simulink model "Model_PID_pitch2010a"  (Simulink 8.9)
settings: Solver=ode45  StartTime=0.0  StopTime=100  RelTol=1e-3  EnableMultiTasking=on
libraries: fuzblock x1
settings Model: Creator=Eng mohammad dradkah  LastModifiedBy=Andres
settings OptimizationCC: ExpressionDepthLimit=2147483647  InitFltsAndDblsToZero=on
settings DebuggingCC: SaveWithParameterizedLinksMsg=none  SignalResolutionControl=TryResolveAllWithWarning  MultiTaskDSMMsg=warning  MultiTaskCondExecSysMsg=none
settings GRTTargetCC: TargetFcnLib=ansi_tfl_tmw.mat  GeneratePreprocessorConditionals=Use local settings

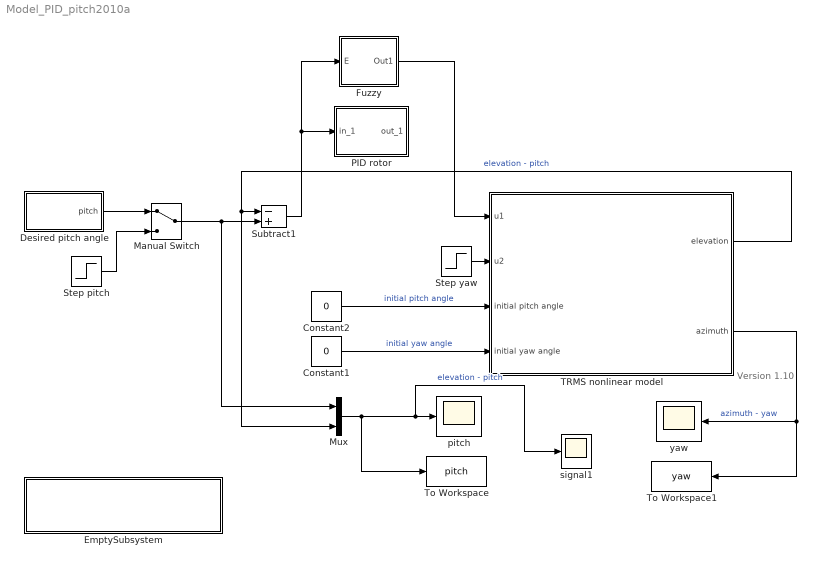
== system Model_PID_pitch2010a ==
  note: Version 1.10
  Constant1 : Constant  Value=0
  Constant2 : Constant  Value=0
  Desired pitch angle : Subsystem
  EmptySubsystem : Subsystem
      mask Display:
      | image(imread('FB-inst-blue2.jpg'))
      | disp('\n\nFeedback Instruments Limited')
  Fuzzy : Subsystem
  Manual Switch : ManualSwitch
  Mux : Mux  Inputs=2
  PID rotor : Subsystem  mask(PID CONTROLLER){KP=3, KI=8, KD=10}
      mask help: PID Main Motor
      mask Display:
      | image(imread('bckg.bmp'))
      | disp('PID')
  Step pitch : Step  Time=0  After=0.4  SampleTime=0
  Step yaw : Step  Time=0  After=0  SampleTime=0
  Subtract1 : Sum  Inputs=-+
  TRMS nonlinear model : Subsystem  mask{I1=6.8e-2, B1psi=6e-3, B2psi=1e-3, a1=0.0135, b1=0.0924, Kgy=0.05, Mfg=0.32, I2=2e-2, B1phi=1e-1, B2phi=1e-3, a2=0.01, b2=0.09}
      mask prompts: I1 "Moment of interia (main motor)"; B1psi "Friction torque (main motor) B1 psi"; B2psi "Friction torque (main motor) B2 psi"; a1 "Static characteristic (main motor) a1"; b1 "Static characteristic (main motor) b1"; Kgy "Parameter Kgy"; Mfg "Moment of gravitation"; I2 "Moment of interia (tail motor)"; B1phi "Friction torque (tail motor) B1 phi"; B2phi "Friction torque (tail motor) B2 phi"; a2 "Static characteristic (tail motor) a2"; b2 "Static characteristic (tail motor) b2"
      mask Display: image(imread('trms.bmp'))
  To Workspace : ToWorkspace  VariableName=pitch  SampleTime=0.1
  To Workspace1 : ToWorkspace  VariableName=yaw  SampleTime=0.1
  pitch : Scope
      mask Display: image(imread('scope.jpg'))
  signal1 : Scope
  yaw : Scope
      mask Display: image(imread('scope.jpg'))
  wires:
  Constant2/1 -> TRMS nonlinear model/3(initial pitch angle)  "initial pitch angle"
  Constant1/1 -> TRMS nonlinear model/4(initial yaw angle)  "initial yaw angle"
  Mux/1 -> To Workspace/1, signal1/1, pitch/1  "elevation - pitch"
  Step yaw/1 -> TRMS nonlinear model/2(u2)
  Desired pitch angle/1(pitch) -> Manual Switch/1
  Step pitch/1 -> Manual Switch/2
  Manual Switch/1 -> Subtract1/2, Mux/1
  TRMS nonlinear model/1(elevation) -> Subtract1/1, Mux/2  "elevation - pitch"
  TRMS nonlinear model/2(azimuth) -> yaw/1, To Workspace1/1  "azimuth - yaw"
  Subtract1/1 -> Fuzzy/1(E), PID rotor/1(in_1)
  Fuzzy/1(Out1) -> TRMS nonlinear model/1(u1)

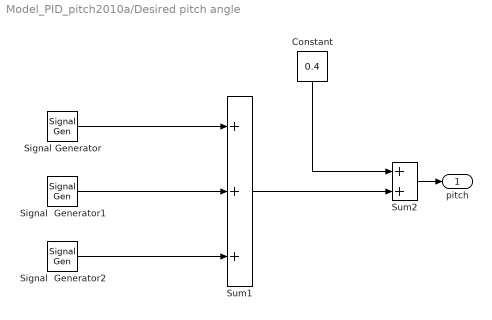
== system Model_PID_pitch2010a/Desired pitch angle ==
  Constant : Constant  Value=0.4
  Signal Generator : SignalGenerator  Amplitude=0.1  Frequency=0.1
  Signal  Generator1 : SignalGenerator  Amplitude=0.1  Frequency=0.05
  Signal  Generator2 : SignalGenerator  Amplitude=0  Frequency=0.02
  Sum1 : Sum  Inputs=+++
  Sum2 : Sum
  pitch : Outport
  wires:
  Signal Generator/1 -> Sum1/1
  Signal  Generator1/1 -> Sum1/2
  Signal  Generator2/1 -> Sum1/3
  Sum2/1 -> pitch/1
  Sum1/1 -> Sum2/2
  Constant/1 -> Sum2/1

== system Model_PID_pitch2010a/EmptySubsystem ==

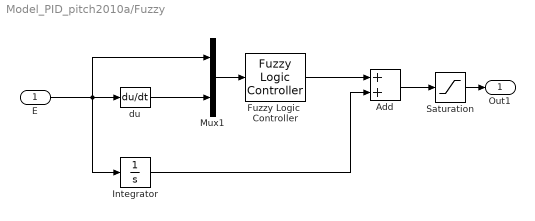
== system Model_PID_pitch2010a/Fuzzy ==
  E : Inport
  Add : Sum
  Fuzzy Logic  Controller : fuzblock/Fuzzy Logic  Controller  fis=FuzzyController
  Integrator : Integrator
  Mux1 : Mux  Inputs=2
  Saturation : Saturate  UpperLimit=2.5  LowerLimit=-2.5
  du : Derivative
  Out1 : Outport
  wires:
  Mux1/1 -> Fuzzy Logic  Controller/1
  E/1 -> Mux1/1, Integrator/1, du/1
  du/1 -> Mux1/2
  Saturation/1 -> Out1/1
  Fuzzy Logic  Controller/1 -> Add/1
  Add/1 -> Saturation/1
  Integrator/1 -> Add/2

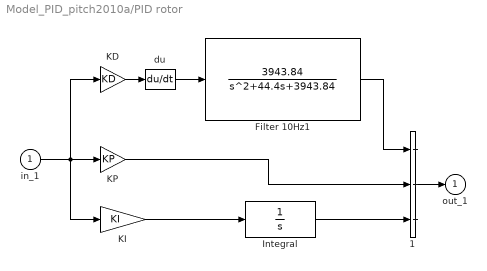
== system Model_PID_pitch2010a/PID rotor ==
  in_1 : Inport
  1 : Sum  Inputs=+++  SaturateOnIntegerOverflow=on  InputSameDT=on  OutDataTypeStr=Inherit: Same as first input
  Filter 10Hz1 : TransferFcn  Numerator=[3943.84]  Denominator=[1 44.4 3943.84]
  Integral : TransferFcn  Denominator=[1 0]
  KD : Gain  Gain=KD  SaturateOnIntegerOverflow=on  OutDataTypeStr=Inherit: Same as input  ParamDataTypeStr=Inherit: Same as input
  KI : Gain  Gain=KI  SaturateOnIntegerOverflow=on  OutDataTypeStr=Inherit: Same as input  ParamDataTypeStr=Inherit: Same as input
  KP : Gain  Gain=KP  SaturateOnIntegerOverflow=on  OutDataTypeStr=Inherit: Same as input  ParamDataTypeStr=Inherit: Same as input
  du : Derivative
  out_1 : Outport  InitialOutput=0
  wires:
  Integral/1 -> 1/3
  KI/1 -> Integral/1
  1/1 -> out_1/1
  du/1 -> Filter 10Hz1/1
  KD/1 -> du/1
  KP/1 -> 1/2
  in_1/1 -> KD/1, KI/1, KP/1
  Filter 10Hz1/1 -> 1/1

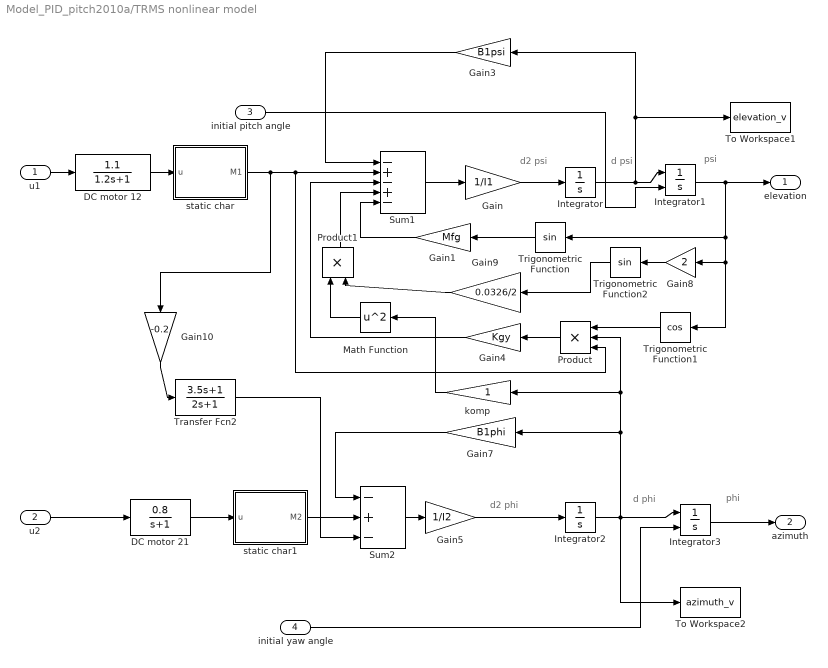
== system Model_PID_pitch2010a/TRMS nonlinear model ==
  note: phi
  note: d phi
  note: d2 phi
  note: psi
  note: d psi
  note: d2 psi
  u1 : Inport
  u2 : Inport  Port=2
  initial pitch angle : Inport  Port=3
  initial yaw angle : Inport  Port=4
  DC motor 12 : TransferFcn  Numerator=[1.1]  Denominator=[1.2 1]
  DC motor 21 : TransferFcn  Numerator=[0.8]  Denominator=[1 1]
  Gain : Gain  Gain=1/I1
  Gain1 : Gain  Gain=Mfg
  Gain10 : Gain  Gain=-0.2
  Gain3 : Gain  Gain=B1psi
  Gain4 : Gain  Gain=Kgy
  Gain5 : Gain  Gain=1/I2
  Gain7 : Gain  Gain=B1phi
  Gain8 : Gain  Gain=2
  Gain9 : Gain  Gain=0.0326/2
  Integrator : Integrator
  Integrator1 : Integrator  InitialConditionSource=external  InitialCondition=0.1
  Integrator2 : Integrator
  Integrator3 : Integrator  InitialConditionSource=external
  Math Function : Math  Operator=square  SaturateOnIntegerOverflow=on
  Product : Product  Inputs=3  RndMeth=Zero
  Product1 : Product  RndMeth=Zero
  Sum1 : Sum  Inputs=-+-+-
  Sum2 : Sum  Inputs=-+-
  To Workspace1 : ToWorkspace  VariableName=elevation_v  SampleTime=-1
  To Workspace2 : ToWorkspace  VariableName=azimuth_v  SampleTime=-1
  Transfer Fcn2 : TransferFcn  Numerator=[3.5 1]  Denominator=[2 1]
  Trigonometric Function : Trigonometry
  Trigonometric Function1 : Trigonometry  Operator=cos
  Trigonometric Function2 : Trigonometry
  komp : Gain
  static char : Subsystem
  static char1 : Subsystem
  elevation : Outport
  azimuth : Outport  Port=2
  wires:
  komp/1 -> Math Function/1
  DC motor 12/1 -> static char/1(u)
  Gain10/1 -> Transfer Fcn2/1
  Math Function/1 -> Product1/1
  Product1/1 -> Sum1/4
  Gain9/1 -> Product1/2
  Trigonometric Function2/1 -> Gain9/1
  Gain8/1 -> Trigonometric Function2/1
  Transfer Fcn2/1 -> Sum2/3
  u2/1 -> DC motor 21/1
  Integrator3/1 -> azimuth/1
  Gain7/1 -> Sum2/1
  Integrator2/1 -> komp/1, Product/2, Gain7/1, To Workspace2/1, Integrator3/1
  Gain5/1 -> Integrator2/1
  Sum2/1 -> Gain5/1
  static char1/1(M2) -> Sum2/2
  DC motor 21/1 -> static char1/1(u)
  Gain4/1 -> Sum1/3
  Product/1 -> Gain4/1
  Trigonometric Function1/1 -> Product/1
  Gain3/1 -> Sum1/1
  static char/1(M1) -> Product/3, Sum1/2, Gain10/1
  Gain1/1 -> Sum1/5
  Trigonometric Function/1 -> Gain1/1
  Integrator1/1 -> elevation/1, Trigonometric Function1/1, Gain8/1, Trigonometric Function/1
  Integrator/1 -> Gain3/1, To Workspace1/1, Integrator1/1
  Gain/1 -> Integrator/1
  Sum1/1 -> Gain/1
  initial pitch angle/1 -> Integrator1/2
  initial yaw angle/1 -> Integrator3/2
  u1/1 -> DC motor 12/1

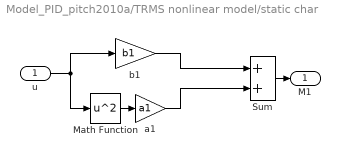
== system Model_PID_pitch2010a/TRMS nonlinear model/static char ==
  u : Inport
  Math Function : Math  Operator=square  SaturateOnIntegerOverflow=on
  Sum : Sum
  a1 : Gain  Gain=a1
  b1 : Gain  Gain=b1
  M1 : Outport
  wires:
  u/1 -> b1/1, Math Function/1
  Math Function/1 -> a1/1
  a1/1 -> Sum/2
  b1/1 -> Sum/1
  Sum/1 -> M1/1

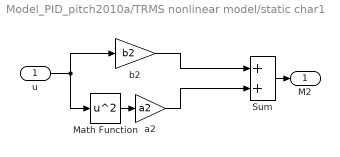
== system Model_PID_pitch2010a/TRMS nonlinear model/static char1 ==
  u : Inport
  Math Function : Math  Operator=square  SaturateOnIntegerOverflow=on
  Sum : Sum
  a2 : Gain  Gain=a2
  b2 : Gain  Gain=b2
  M2 : Outport
  wires:
  Sum/1 -> M2/1
  b2/1 -> Sum/1
  a2/1 -> Sum/2
  Math Function/1 -> a2/1
  u/1 -> Math Function/1, b2/1
